simulink model "polydezim_2_"  (Simulink 7.8)
settings: Solver=FixedStepDiscrete  SolverMode=SingleTasking  StartTime=0.0  StopTime=10.0  RelTol=1e-3
values from neighbouring files (symbols this model uses):
  h = firpm(64,f,m)    [CFIR_1.m]    (also in adapt_filter1.m = adaptfilt.lms(ni,mu); adapt_filter2.m = adaptfilt.blms(ni,mu,1,36); adaptiv_2.m = [1 2 3 4 5 6 7 8 9 10]; adaptiv_3.m = [1 2 3 4 5 6 7 8 9 10])
  M = 2    [CFIR_1.m]    (also in block_lms_.m = 16; cic_dezim1.m = ',num2str(M),'; cic_dezim1_.m = ',num2str(M),     '; cic_dezim2.m = ',num2str(M),')
  Ts = 1/fs    (= 6.25e-05)    [G722_1.m]    (also in adaptiv_2.m = 0.001; adaptiv_3.m = 0.001; adaptiv_4.m = 0.001; adaptiv_5.m = 0.001)
undefined symbols (not defined in the file or in its folder): g
libraries: dspsigops x2, dspobslib x1
settings Model: Creator=svenhoffmann  LastModifiedBy=josef  ExtModeAutoUpdateStatusClock=off
settings DataIOCC: SignalLoggingName=sigsOut
settings OptimizationCC: InitFltsAndDblsToZero=on
settings DebuggingCC: SaveWithParameterizedLinksMsg=none  SignalResolutionControl=TryResolveAllWithWarning  SolverPrmCheckMsg=none  MultiTaskDSMMsg=warning  MultiTaskCondExecSysMsg=none  FcnCallInpInsideContextMsg=Use local settings  StrictBusMsg=None
settings HardwareCC: TargetUnknown=on
settings RTWCC: IncludeERTFirstTime=on
settings GRTTargetCC: TargetFcnLib=ansi_tfl_tmw.mat

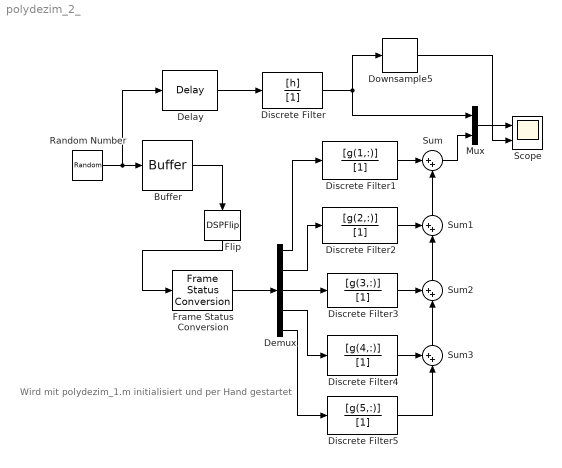
== system polydezim_2_ ==
  note: Wird mit polydezim_1.m initialisiert
      | und per Hand gestartet
  Buffer : Buffer  N=M
  Delay : dspsigops/Delay  InputProcessing=Inherited (this choice will be removed - see release notes)  dly_unit=Samples  delay=1  ic_detail=off  dif_ic_for_ch=off  dif_ic_for_dly=off  ic=0  reset_popup=None
  Demux : Demux  Outputs=M
  Discrete Filter : DiscreteFilter  Numerator=[h]  Denominator=[1]  SampleTime=Ts
  Discrete Filter1 : DiscreteFilter  Numerator=[g(1,:)]  Denominator=[1]  SampleTime=Ts*5
  Discrete Filter2 : DiscreteFilter  Numerator=[g(2,:)]  Denominator=[1]  SampleTime=Ts*5
  Discrete Filter3 : DiscreteFilter  Numerator=[g(3,:)]  Denominator=[1]  SampleTime=Ts*5
  Discrete Filter4 : DiscreteFilter  Numerator=[g(4,:)]  Denominator=[1]  SampleTime=Ts*5
  Discrete Filter5 : DiscreteFilter  Numerator=[g(5,:)]  Denominator=[1]  SampleTime=Ts*5
  Downsample5 : dspsigops/Downsample  N=5  phase=0  InputProcessing=Inherited (this choice will be removed - see release notes)  RateOptions=Enforce single-rate processing  smode=Allow multirate  fmode=Maintain input frame size  ic=0
  Flip : DSPFlip
  Frame Status Conversion : dspobslib/Frame Status Conversion  growRefPort=off  outframe=Sample-based
  Mux : Mux  Inputs=2
  Random Number : RandomNumber  SampleTime=Ts
  Scope : Scope  NumInputPorts=2
      settings: YMin=-5~-5  YMax=5~5
  Sum : Sum  Inputs=|++  SaturateOnIntegerOverflow=on
  Sum1 : Sum  Inputs=++|  SaturateOnIntegerOverflow=on
  Sum2 : Sum  Inputs=++|  SaturateOnIntegerOverflow=on
  Sum3 : Sum  Inputs=++|  SaturateOnIntegerOverflow=on
  wires:
  Discrete Filter/1 -> Mux/1, Downsample5/1
  Mux/1 -> Scope/1
  Discrete Filter2/1 -> Sum1/1
  Sum1/1 -> Sum/2
  Sum2/1 -> Sum1/2
  Discrete Filter4/1 -> Sum3/1
  Sum3/1 -> Sum2/2
  Discrete Filter5/1 -> Sum3/2
  Discrete Filter1/1 -> Sum/1
  Discrete Filter3/1 -> Sum2/1
  Random Number/1 -> Buffer/1, Delay/1
  Demux/1 -> Discrete Filter1/1
  Demux/2 -> Discrete Filter2/1
  Demux/3 -> Discrete Filter3/1
  Demux/4 -> Discrete Filter4/1
  Demux/5 -> Discrete Filter5/1
  Frame Status Conversion/1 -> Demux/1
  Buffer/1 -> Flip/1
  Flip/1 -> Frame Status Conversion/1
  Downsample5/1 -> Scope/2
  Sum/1 -> Mux/2
  Delay/1 -> Discrete Filter/1
